simulink model "RLModel"  (R2024b)
settings: Solver=VariableStepAuto  StartTime=0.0  StopTime=Tf  RelTol=1e-3  AbsTol=1e-3  EnableMultiTasking=on
InitFcn:
  | ModelParameters;
values from neighbouring files (symbols this model uses):
  foot_height = 0.05    [ModelParameters.m]
  foot_length = 0.3    [ModelParameters.m]
  foot_width = 0.2    [ModelParameters.m]
  init_height = plane_height/2 + foot_height + shank_height + thigh_height + 0.5*torso_height    (= 1.65)    [ModelParameters.m]
  left = [0,          0,          0]    [ModelParameters.m]
  max_torque = 1000    [ModelParameters.m]
  plane_height = 0.2    [ModelParameters.m]
  right = [0,          0,          0]    [ModelParameters.m]
  shank_height = 0.5    [ModelParameters.m]
  shank_length = 0.2    [ModelParameters.m]
  shank_width = 0.2    [ModelParameters.m]
  Tf = 10.0    (= 10)    [ModelParameters.m]
  thigh_height = 0.5    [ModelParameters.m]
  thigh_length = 0.2    [ModelParameters.m]
  thigh_width = 0.2    [ModelParameters.m]
  torso_height = 1.0    (= 1)    [ModelParameters.m]
  torso_length = 0.2    [ModelParameters.m]
  torso_width = 0.5    [ModelParameters.m]
  Ts = 0.025    [ModelParameters.m]
undefined symbols (not defined in the file or in its folder): X, Y, Z
libraries: sm_lib x62, nesl_utility x25, rllib x1, simulink x1
(part 3 of 3)

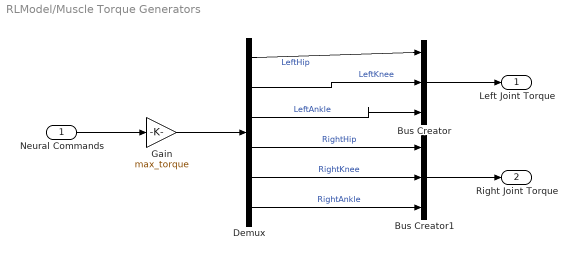
== system RLModel/Muscle Torque Generators ==
  Neural Commands : Inport
  Bus Creator : BusCreator  Inputs=3
  Bus Creator1 : BusCreator  Inputs=3
  Demux : Demux  Outputs=6
  Gain : Gain  Gain=max_torque
  Left Joint Torque : Outport
  Right Joint Torque : Outport  Port=2
  wires:
  Demux/1 -> Bus Creator/1  "LeftHip"
  Bus Creator/1 -> Left Joint Torque/1
  Bus Creator1/1 -> Right Joint Torque/1
  Demux/2 -> Bus Creator/2  "LeftKnee"
  Demux/3 -> Bus Creator/3  "LeftAnkle"
  Demux/4 -> Bus Creator1/1  "RightHip"
  Demux/5 -> Bus Creator1/2  "RightKnee"
  Demux/6 -> Bus Creator1/3  "RightAnkle"
  Neural Commands/1 -> Gain/1
  Gain/1 -> Demux/1

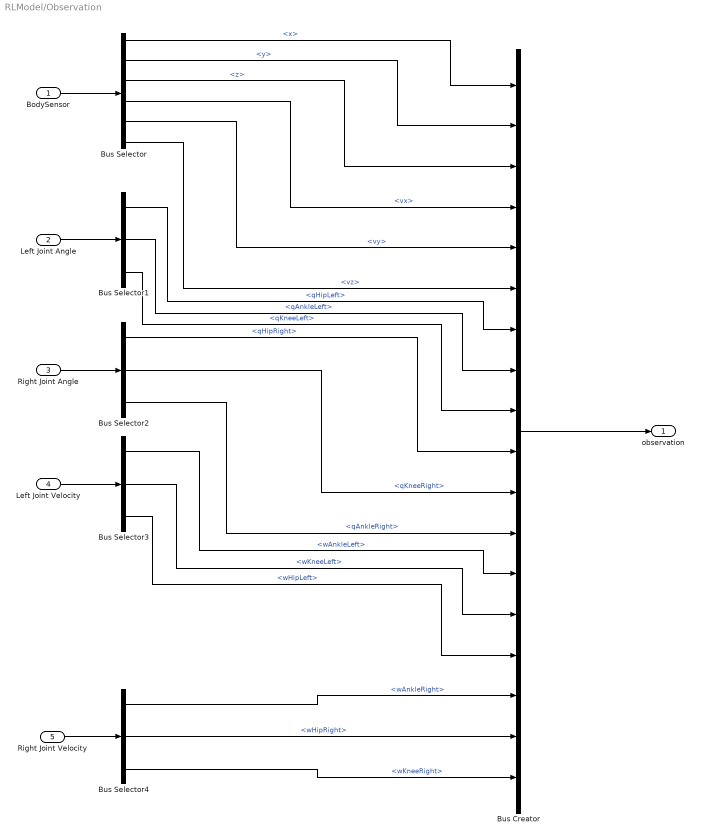
== system RLModel/Observation ==
  BodySensor : Inport
  Left Joint Angle : Inport  Port=2
  Right Joint Angle : Inport  Port=3
  Left Joint Velocity : Inport  Port=4
  Right Joint Velocity : Inport  Port=5
  Bus Creator : BusCreator  Inputs=18
  Bus Selector : BusSelector  OutputSignals=x,y,z,vx,vy,vz
  Bus Selector1 : BusSelector  OutputSignals=qHipLeft,qAnkleLeft,qKneeLeft
  Bus Selector2 : BusSelector  OutputSignals=qHipRight,qKneeRight,qAnkleRight
  Bus Selector3 : BusSelector  OutputSignals=wAnkleLeft,wKneeLeft,wHipLeft
  Bus Selector4 : BusSelector  OutputSignals=wAnkleRight,wHipRight,wKneeRight
  observation : Outport
  wires:
  BodySensor/1 -> Bus Selector/1
  Left Joint Angle/1 -> Bus Selector1/1
  Right Joint Angle/1 -> Bus Selector2/1
  Left Joint Velocity/1 -> Bus Selector3/1
  Right Joint Velocity/1 -> Bus Selector4/1
  Bus Selector/1 -> Bus Creator/1  "<x>"
  Bus Selector/2 -> Bus Creator/2  "<y>"
  Bus Selector/3 -> Bus Creator/3  "<z>"
  Bus Selector/4 -> Bus Creator/4  "<vx>"
  Bus Selector/5 -> Bus Creator/5  "<vy>"
  Bus Selector/6 -> Bus Creator/6  "<vz>"
  Bus Selector1/1 -> Bus Creator/7  "<qHipLeft>"
  Bus Selector1/2 -> Bus Creator/8  "<qAnkleLeft>"
  Bus Selector1/3 -> Bus Creator/9  "<qKneeLeft>"
  Bus Selector2/1 -> Bus Creator/10  "<qHipRight>"
  Bus Selector2/2 -> Bus Creator/11  "<qKneeRight>"
  Bus Selector2/3 -> Bus Creator/12  "<qAnkleRight>"
  Bus Selector3/1 -> Bus Creator/13  "<wAnkleLeft>"
  Bus Selector3/2 -> Bus Creator/14  "<wKneeLeft>"
  Bus Selector3/3 -> Bus Creator/15  "<wHipLeft>"
  Bus Selector4/1 -> Bus Creator/16  "<wAnkleRight>"
  Bus Selector4/2 -> Bus Creator/17  "<wHipRight>"
  Bus Selector4/3 -> Bus Creator/18  "<wKneeRight>"
  Bus Creator/1 -> observation/1

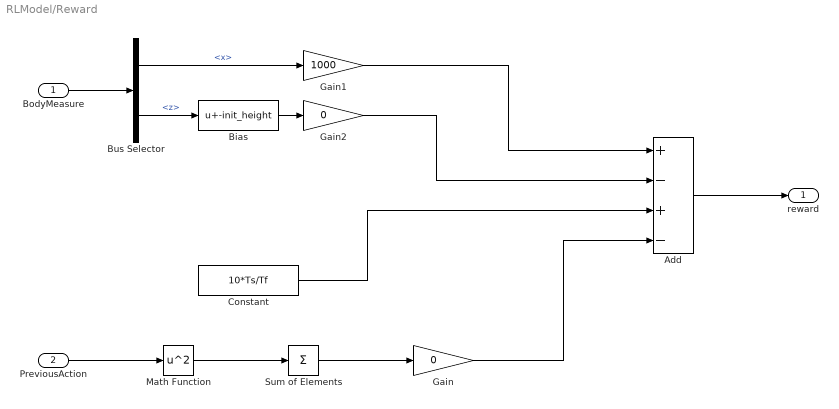
== system RLModel/Reward ==
  BodyMeasure : Inport
  PreviousAction : Inport  Port=2
  Add : Sum  Inputs=+-+-
  Bias : Bias  Bias=-init_height  SaturateOnIntegerOverflow=off
  Bus Selector : BusSelector  OutputSignals=x,z
  Constant : Constant  Value=10*Ts/Tf
  Gain : Gain  Gain=0
  Gain1 : Gain  Gain=1000
  Gain2 : Gain  Gain=0
  Math Function : Math  Operator=square
  Sum of Elements : Sum  Inputs=+
  reward : Outport
  wires:
  PreviousAction/1 -> Math Function/1
  Math Function/1 -> Sum of Elements/1
  Sum of Elements/1 -> Gain/1
  BodyMeasure/1 -> Bus Selector/1
  Bias/1 -> Gain2/1
  Gain1/1 -> Add/1
  Gain2/1 -> Add/2
  Constant/1 -> Add/3
  Gain/1 -> Add/4
  Add/1 -> reward/1
  Bus Selector/1 -> Gain1/1  "<x>"
  Bus Selector/2 -> Bias/1  "<z>"

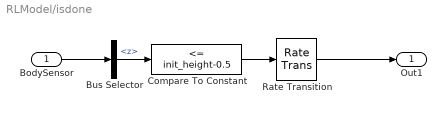
== system RLModel/isdone ==
  BodySensor : Inport
  Bus Selector : BusSelector  OutputSignals=z
  Compare To Constant : simulink/Logic and Bit Operations/Compare To Constant  relop=<=  const=init_height-0.5  OutDataTypeStr=boolean
  Rate Transition : RateTransition
  Out1 : Outport
  wires:
  BodySensor/1 -> Bus Selector/1
  Bus Selector/1 -> Compare To Constant/1  "<z>"
  Rate Transition/1 -> Out1/1
  Compare To Constant/1 -> Rate Transition/1
